simulink model "levitron_ctrl"  (Simulink 7.1)
settings: Solver=ode45  StartTime=0.0  StopTime=10.0  RelTol=1e-3
settings Model: Creator=volgy  LastModifiedBy=volgy

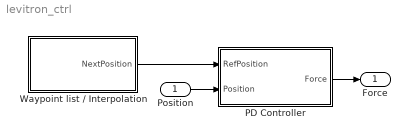
== system levitron_ctrl ==
  Position : Inport  PortDimensions=1  DataType=single  OutDataType=sfix(16)  OutScaling=2^0  OutDataTypeStr=single
  PD Controller : Subsystem  AncestorBlock=levitron_lib/PD Controller
  Waypoint list / Interpolation : Subsystem  AncestorBlock=levitron_lib/Waypoint list // Interpolation
  Force : Outport  PortDimensions=1  DataType=single  OutDataType=sfix(16)  OutScaling=2^0  OutDataTypeStr=single
  wires:
  Waypoint list / Interpolation/1(NextPosition) -> PD Controller/1(RefPosition)
  Position/1 -> PD Controller/2(Position)
  PD Controller/1(Force) -> Force/1

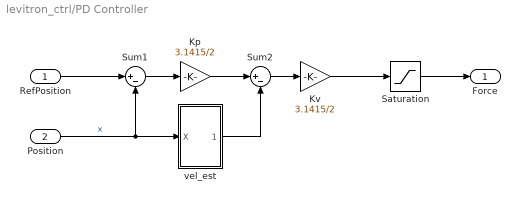
== system levitron_ctrl/PD Controller ==
  RefPosition : Inport
  Position : Inport  Port=2
  Kp : Gain  Gain=3.1415/2  ParameterDataType=sfix(16)  ParameterScaling=2^0  OutDataType=sfix(16)  OutScaling=2^0
  Kv : Gain  Gain=3.1415/2  ParameterDataType=sfix(16)  ParameterScaling=2^0  OutDataType=sfix(16)  OutScaling=2^0
  Saturation : Saturate  UpperLimit=100  LowerLimit=0  OutDataType=sfix(16)  OutScaling=2^0
  Sum1 : Sum  Inputs=|+-  OutDataType=sfix(16)  OutScaling=2^0
  Sum2 : Sum  Inputs=|+-  OutDataType=sfix(16)  OutScaling=2^0
  vel_est : Subsystem
  Force : Outport
  wires:
  Position/1 -> vel_est/1(X), Sum1/2  "x"
  RefPosition/1 -> Sum1/1
  Saturation/1 -> Force/1
  Sum1/1 -> Kp/1
  Kp/1 -> Sum2/1
  vel_est/1(V_est) -> Sum2/2
  Sum2/1 -> Kv/1
  Kv/1 -> Saturation/1

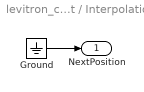
== system levitron_ctrl/Waypoint list / Interpolation ==
  Ground : Ground
  NextPosition : Outport  PortDimensions=1  SampleTime=1  DataType=single  OutDataTypeStr=single
  wires:
  Ground/1 -> NextPosition/1

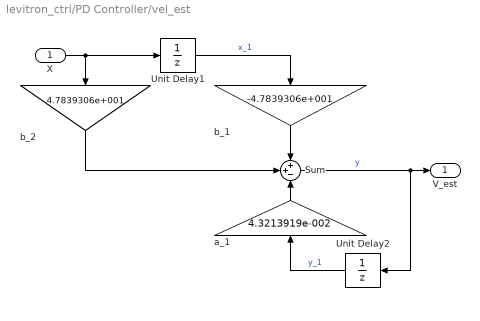
== system levitron_ctrl/PD Controller/vel_est ==
  X : Inport
  Sum : Sum  Inputs=++-  AccumDataTypeStr=single  OutDataType=sfix(16)  OutScaling=2^0
  Unit Delay1 : UnitDelay  SampleTime=-1
  Unit Delay2 : UnitDelay  Orientation=left  SampleTime=-1
  a_1 : Gain  Orientation=up  Gain=4.3213919e-002  ParameterDataType=sfix(16)  ParameterScaling=2^0  OutDataTypeMode=single  OutDataType=sfix(16)  OutScaling=2^0  OutDataTypeStr=single
  b_1 : Gain  Orientation=down  Gain=-4.7839306e+001  ParameterDataType=sfix(16)  ParameterScaling=2^0  OutDataTypeMode=single  OutDataType=sfix(16)  OutScaling=2^0  OutDataTypeStr=single
  b_2 : Gain  Orientation=down  Gain=4.7839306e+001  ParameterDataType=sfix(16)  ParameterScaling=2^0  OutDataTypeMode=single  OutDataType=sfix(16)  OutScaling=2^0  OutDataTypeStr=single
  V_est : Outport
  wires:
  Unit Delay1/1 -> b_1/1  "x_1"
  b_1/1 -> Sum/1
  b_2/1 -> Sum/2
  Sum/1 -> Unit Delay2/1, V_est/1  "y"
  a_1/1 -> Sum/3
  Unit Delay2/1 -> a_1/1  "y_1"
  X/1 -> b_2/1, Unit Delay1/1
